simulink model "RedCrane_Topology_Merged"  (R2024b)
settings: Solver=VariableStepAuto  StartTime=0.0  StopTime=1  RelTol=1e-4
model workspace (MATLAB code in the model file):
  | %% Geometric properties
  | 
  | %Mounting
  | L_M = 1; %m
  | W_M = 1; %m
  | H_M = 1; %m
  | eta_M = 0; %m
  | zeta_M = -0.5; %m
  | beta_M = 0; %m
  | 
  | %Ground
  | L_ground = 6; %m
  | W_ground = 4; %m
  | H_ground = 0.01; %m
  | eta_ground = 1.5; %m
  | zeta_ground = -0.5; %m
  | beta_ground = 0; %m
  | 
  | 
  | %Basic geometry width
  | w0 = 0.07;
  | w1 = w0/4;
  | l_RJ = 0.277; %2.1*w0;
  | r_RJ = 0.030;
  | 
  | %Column geometry
  | L_Column = 1.5655; %2;
  | eta_B = -0.25;
  | zeta_B = L_Column;
  | eta_D = -0.365; %0.25;
  | zeta_D = 1.4805; %1.5;
  | eta_J = 0.200; % 0.25;
  | zeta_J = 0.1195; %0.25;
  | 
  | %Column - main boom link
  | l_DE = 0.490; % 0.5;
  | l_FE = 0.170; % 0.4;
  | 
  | %Main boom geometry
  | L_Mboom = 2.400; % 2;
  | eta_C = 2.400; % 2;
  | zeta_C = 0.070; % 0.25;
  | eta_F = 0.340; % 0.6;
  | zeta_F = 0.010; % -0.25;
  | eta_G = 2.365; % 1.75;
  | zeta_G = 0.235; % -0.25;
  | eta_K = 0.750; % 1;
  | zeta_K = 0.045; % -0.25;
  | 
  | %Main boom-knuckle boom link
  | l_GH = 0.490; % 0.5;
  | l_IH = 0.220; % 0.4;
  | 
  | %Knuckle boom geometry
  | L_Kboom = 2.429; % 2;
  | eta_I = 0.280; % 0.5;
  | zeta_I = 0.005; % -0.25;
  | eta_TP = L_Kboom;
  | zeta_TP = 0;
  | 
  | % Winch
  | r_W = 0.205/2;
  | L_W = 0.191;
  | eta_W = 0.28722;
  | zeta_W = -0.29926;
  | beta_W = -0.335;
  | 
  | %Mounting plate
  | eta_MP = -0.0249;
  | zeta_MP = -0.17479;
  | beta_MP = 0;
  | 
  | % Pulley
  | r_P = 0.210/2; % Radius pulley
  | eta_P = 2.140;
  | zeta_P = -0.0506;
  | beta_P = -0.0;
  | 
  | %Rull
  | r_RO = 0.055/2; % Radius rull over
  | r_RU = 0.046/2; % Radius rull under
  | eta_RO = 0.306;
  | zeta_RO = 0.12510;
  | 
  | %% Mass properties (Mass and center of mass)
  | 
  | column_mass = 239.4; % kg
  | column_COM = [-0.1007, 0.0001, 0.4351]; % m
  | 
  | MainBoom_mass = 216.5; % kg
  | MainBoom_COM = [1.134, 0.1674, -0.0018]; % m
  | 
  | KnuckleBoom_mass = 842.2; % kg
  | KnuckleBoom_COM = [0.9806, 0.1814, -0.2939]; % m
  | 
  | % Dogbone
  | E2F_mass = 7.076*2; % kg
  | E2F_COM = [0.0817, 0, 0]; % m
  | 
  | D2E_mass = 6.426*2; % kg
  | D2E_COM = [0.245, 0, 0]; % m
  | 
  | G2H_mass = 6.426*2; % kg
  | G2H_COM = [0.245, 0, 0]; % m
  | 
  | H2I_mass = 22.05; % kg
  | H2I_COM = [0.1206, 0, 0]; % m
  | 
  | % Main cylinder
  | MC_bottom_mass = 57.9561; % kg
  | MC_bottom_COM = [0.0081, -0.001, 0.4125]; % m
  | 
  | MC_rod_mass = 43.93; % kg
  | MC_rod_COM = [0, 0, -0.4290]; % m
  | 
  | % Knuckle cylinder
  | KC_bottom_mass = 55.7738; % kg
  | KC_bottom_COM = [0.0038, 0.0022, 0.4468]; % m
  | 
  | KC_rod_mass = 45.8854; % kg
  | KC_rod_COM = [0, 0, -0.4694]; % m
  | 
  | % Winch
  | Winch_mass = 54; % kg
  | Winch_COM = [0, 0, 0]; % m
  | 
  | 
  | 
  | %% Inertia properties (Moments of inertia and products of inertia)
  | 
  | column_MOI = [109, 114, 9.009]; % kg*m^2
  | column_POI = [0.0319, -21.59, -0.0113]; % kg*m^2
  | 
  | MainBoom_MOI = [6.5, 160.3, 160]; % kg*m^2
  | MainBoom_POI = [0.0666, 0.1093, 8.016]; % kg*m^2
  | 
  | KnuckleBoom_MOI = [31.75, 566.3, 573.1]; % kg*m^2
  | KnuckleBoom_POI = [-0.0237, -11.42, 9.588]; % kg*m^2
  | 
  | % Dogbone
  | E2F_MOI = [0.0111, 0.0546, 0.0587]; % kg*m^2
  | E2F_POI = [0, -0.0089, 0]; % kg*m^2
  | 
  | D2E_MOI = [0.0069, 0.2419, 0.2485]; % kg*m^2
  | D2E_POI = [0, 0, 0]; % kg*m^2
  | 
  | G2H_MOI = [0.0069, 0.2419, 0.2485]; % kg*m^2
  | G2H_POI = [0, 0, 0]; % kg*m^2
  | 
  | H2I_MOI = [0.2636, 0.4184, 0.1901]; % kg*m^2
  | H2I_POI = [0, 0, 0]; % kg*m^2
  | 
  | 
  | % Main cylinder
  | MC_bottom_MOI = [7.2059, 7.2304, 0.3979]; % kg*m^2
  | MC_bottom_POI = [-0.0126, -0.1802, 0.0002]; % kg*m^2
  | 
  | MC_rod_MOI = [6.0014, 5.9633, 0.1401]; % kg*m^2
  | MC_rod_POI = [0, -0.0001, 0]; % kg*m^2
  | 
  | % Knuckle cylinder
  | KC_bottom_MOI = [8.3780, 8.3476, 0.3607]; % kg*m^2
  | KC_bottom_POI = [-0.0119, -0.1037, 0.0033]; % kg*m^2
  | 
  | KC_rod_MOI = [7.4245, 7.3864, 0.1401]; % kg*m^2
  | KC_rod_POI = [0, -0.0001, 0]; % kg*m^2
  | 
  | % Winch
  | I_W_xx = (1/4)*Winch_mass*r_W^2 + (1/12)*Winch_mass*L_W^2;
  | I_W_yy = (1/4)*Winch_mass*r_W^2 + (1/12)*Winch_mass*L_W^2;
  | I_W_zz = (1/2)*Winch_mass*r_W^2;
  | 
  | Winch_MOI = [I_W_xx, I_W_yy, I_W_zz]; % kg*m^2
  | Winch_POI = [0, 0, 0]; % kg*m^2
  | 
  | 
  | 
  | 
  | %% Hydraulics
  | 
  | %-------------Cylinder---------------------
  | 
  | % Main cylinder
  | D_piston_mc = 160; %mm dimater of piston side
  | L_piston_mc = 65; %66.2;%mm length from joint to buttom of piston side
  | D_rod_mc = 100; %mm diamter of cylinder rod
  | L_rod_mc = 978; %990;%mm length from bottom of rod to joint
  | A_piston_mc = pi/4*D_piston_mc^2; % mm^2 area of piston side
  | A_rod_mc = pi/4*D_rod_mc^2; % mm^2 area of rod
  | A_rodside_mc = A_piston_mc-A_rod_mc; % mm^2 area of rod side
  | L_barrel_mc = 945-L_piston_mc; %mm
  | stroke_mc = 0.75; %m
  | initial_pos_main = 0.3; %m
  | initial_Pa_main = 17;%Bar
  | 
  | % Knuckle cylinder
  | D_piston_kc = 150; %mm dimater of piston side
  | L_piston_kc = 65; %66.2;%mm length from joint to buttom of piston side
  | D_rod_kc = 100; %mm diamter of cylinder rod
  | L_rod_kc = 1089.5; %1105.5;%mm length from bottom of rod to joint
  | A_piston_kc = pi/4*D_piston_kc^2; % mm^2 area of piston side
  | A_rod_kc = pi/4*D_rod_kc^2; % mm^2 area of rod
  | A_rodside_kc = A_piston_kc-A_rod_kc; % mm^2 area of rod side
  | L_barrel_kc = 1050-L_piston_kc; %mm
  | stroke_kc = 0.85; %m
  | initial_pos_knuckle = 0.4; %m
  | initial_Pa_knuckle = 1;%Bar
  | initial_Pb_knuckle = 67;%Bar
  | 
  | % winch
  | poly_b = [1.762740809095876e+02,-44.442169999547330];
  | poly_c = [1.901177983521692e+02,-1.484122102902541e+02];
  | angle_b = poly_b(1)*initial_pos_main + poly_b(2);
  | angle_c = poly_c(1)*initial_pos_knuckle + poly_c(2);
  | angle_w = -90 - angle_c - angle_b;
  | 
  | %Motor
  | DM = 200; %Displacement cm^3/rev
  | GR = 5.04; % Gear ratio 1:5,04
  | 
  | 
  | % ------------------CBV-------------------
  | 
  | % Main
  | pCr_main = 25;%Bar
  | dpopen_main = 300;%Bar
  | 
  | % Knuckle
  | alpha = 4.25;
  | pCr_ka = 211;%Bar
  | dpopen_ka = 300;%Bar
  | pCr_kb = 211;%Bar
  | dpopen_kb = 300;%Bar
  | 
  | %-------------------DCV-----------------------
  | Cd = 0.64;
  | Q_rat = 30/6e4;
  | dp_2 = 6e5;
  | dp_1 = 1e5;
  | roh = 850;
  | 
  | %main dcv
  | dead_up_m = 0.175;
  | dead_down_m = 0.155;
  | 
  | %knuckle dcv
  | dead_up_k = 0.18;
  | dead_down_k = 0.205;
  | 
  | Ad2 = Q_rat/(Cd*sqrt(2/roh*dp_2))*1e6; %mm
  | Ad1_1 = Q_rat/(Cd*sqrt(2/roh*dp_1))*1e6;
  | Ad1_0 = Q_rat/(Cd*sqrt(2/roh*dp_1))*1e6*0;
  | 
  | Ad1_mup = Q_rat/(Cd*sqrt(2/roh*dp_1))*1e6*dead_up_m;
  | Ad1_mdown = Q_rat/(Cd*sqrt(2/roh*dp_1))*1e6*dead_down_m;
  | Ad1_kup = Q_rat/(Cd*sqrt(2/roh*dp_1))*1e6*dead_up_k;
  | Ad1_kdown = Q_rat/(Cd*sqrt(2/roh*dp_1))*1e6*dead_down_k;
undefined symbols (not defined in the file): X, Y, Z
libraries: sm_lib x171, fl_lib x64, nesl_utility x47, SimscapeFluids_lib x27, sdl_lib x1
(part 8 of 8)

== matlab function RedCrane_Topology_Merged/Knuckle cylinder/Subsystem3/CBV_opening_A ==
  data: pB input; uCBV output; pAm input; pA input; pCr_ka parameter; dpopen_ka parameter; alpha parameter
function uCBV = fcn(pB,pAm,pA,pCr_ka, dpopen_ka, alpha)

uCBV = (alpha*pB + pAm - pCr_ka - (alpha + 1)*pA)/dpopen_ka;
%uCBV = (alpha*pB + pAm - pCr)/dpopen; %vented
%uCBV = 0.25;
if uCBV < 0
    uCBV = 0;
elseif uCBV > 1
    uCBV = 1;
end

== matlab function RedCrane_Topology_Merged/Main cylinder/Subsystem3/CBV_opening_A ==
  data: pB input; uCBV output; pA input; pCr_main parameter; dpopen_main parameter
function uCBV = fcn(pB,pA,pCr_main, dpopen_main)
% uCBV = (alpha*pB + pAm - pCr - (alpha + 1)*pA)/dpopen;
uCBV = (pB - pCr_main- pA)/dpopen_main; %vented
%uCBV = 0.25;
if uCBV < 0
    uCBV = 0;
elseif uCBV > 1
    uCBV = 1;
end

== matlab function RedCrane_Topology_Merged/Main cylinder/Subsystem2/uAT ==
  data: U input; u output; dead_up_m parameter; dead_down_m parameter
function u = fcn(U,dead_up_m, dead_down_m)
if U < -dead_up_m
    u=0;
elseif U <= 0
    u = dead_down_m-abs(U);
elseif U <= dead_down_m
    u = dead_down_m;
elseif U >dead_down_m
    u= (U-dead_down_m)/(1-dead_down_m)+dead_down_m;
else
    u = 0;
end

== matlab function RedCrane_Topology_Merged/Main cylinder/Subsystem2/uBT ==
  data: U input; u output; dead_up_m parameter; dead_down_m parameter
function u = fcn(U,dead_up_m, dead_down_m)
if U < -dead_down_m
    u=0;
elseif U <= 0
    u = dead_up_m-abs(U);
elseif U <= dead_up_m
    u = dead_up_m;
elseif U >dead_up_m
    u= (U-dead_up_m)/(1-dead_up_m)+dead_up_m;
else
    u = 0;
end
